simulink model "position_control_model"  (R2018b)
settings: Solver=VariableStepAuto  StartTime=0.0  StopTime=10.0  RelTol=1e-3
values from neighbouring files (symbols this model uses):
  GP_den = [1 1021 4845 0]    [lecture_control_system_designer.m]
  GP_num = [46163]    [lecture_control_system_designer.m]
settings Model: Creator=Christopher  LastModifiedBy=chris

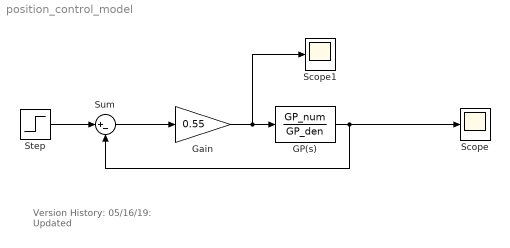
== system position_control_model ==
  note: Version History:
      | 05/16/19: Updated
  GP(s) : TransferFcn  Numerator=GP_num  Denominator=GP_den
  Gain : Gain  Gain=0.55
  Scope : Scope
  Scope1 : Scope
  Step : Step  SampleTime=0
  Sum : Sum  Inputs=|+-
  wires:
  Gain/1 -> Scope1/1, GP(s)/1
  GP(s)/1 -> Sum/2, Scope/1
  Sum/1 -> Gain/1
  Step/1 -> Sum/1
